simulink model "State_Feedback_Linear_ROS"  (R2022b)
settings: Solver=FixedStepAuto  StartTime=0.0  StopTime=128  FixedStep=0.02  RelTol=1e-3
undefined symbols (not defined in the file): unicycle, X, Y
libraries: robotlib x3, simulink_extras x2
settings Model: PauseTimes=14.13  Creator=Musta  LastModifiedBy=mustacchim
settings OptimizationCC: EnhancedBackFolding=on  PassReuseOutputArgsAs=Individual arguments  ZeroExternalMemoryAtStartup=off  ZeroInternalMemoryAtStartup=off  MaxStackSize=64  OptimizeBlockOrder=speed  DifferentSizesBufferReuse=on  OptimizationCustomize=off  EfficientTunableParamExpr=on
settings DebuggingCC: ParameterTunabilityLossMsg=error
settings HardwareCC: ProdBitPerPointer=32  ProdBitPerSizeT=32  ProdBitPerPtrDiffT=32  ProdLargestAtomicFloat=None  ProdIntDivRoundTo=Undefined  ProdEndianess=Unspecified  ProdWordSize=32  ProdHWDeviceType=Generic->Unspecified (assume 32-bit Generic)
settings SFSimCC: MATLABDynamicMemAlloc=off
settings RTWCC: Description=Embedded Coder  SystemTargetFile=ert.tlc  HardwareBoard=Robot Operating System (ROS)  TLCOptions="-aInlineSetEventsForThisBaseRateFcn=TLC_FALSE -aSuppressMultiTaskScheduler=TLC_FALSE  -aRateBasedStepFcn=0"  TemplateMakefile=ert_default_tmf  Toolchain=Catkin  TargetLang=C++
settings CodeAppCC: ForceParamTrailComments=on  IgnoreCustomStorageClasses=off  OperatorAnnotations=on  SimulinkDataObjDesc=on  SFDataObjDesc=on  InsertBlockDesc=on

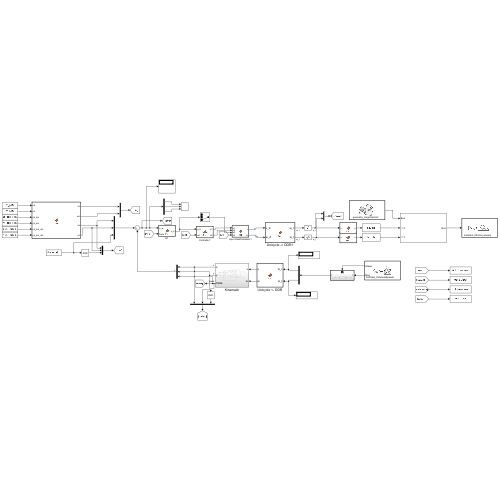
[thumbnail: Simulink's stored preview of the top-level diagram]
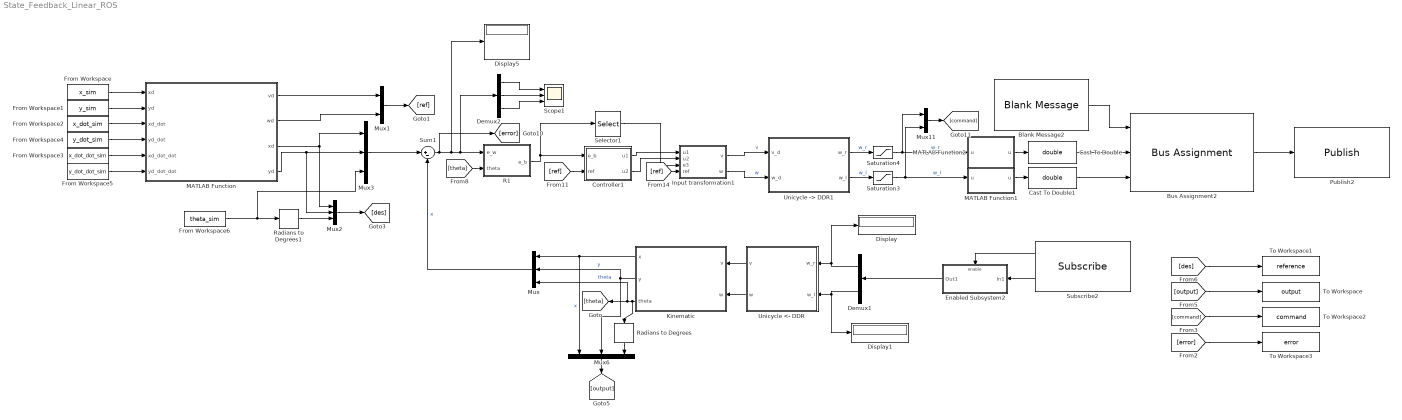
== system State_Feedback_Linear_ROS ==
  Blank Message2 : robotlib/Blank Message  messageClass=Message  entityType=geometry_msgs/Vector3  messageType=geometry_msgs/Vector3  SampleTime=0.02  legacyBusStruct=off
      settings: LibrarySourceBlock=roslib/ROS/Blank Message
  Bus Assignment2 : BusAssignment  AssignedSignals=X,Y
  Cast To Double : DataTypeConversion  OutDataTypeStr=double  SaturateOnIntegerOverflow=off  RndMeth=Floor
  Cast To Double1 : DataTypeConversion  OutDataTypeStr=double  SaturateOnIntegerOverflow=off  RndMeth=Floor
  Controller1 : MATLAB Function  TreatAsAtomicUnit=on
  Demux1 : Demux  Outputs=2
  Demux2 : Demux  Outputs=3
  Display : Display
  Display1 : Display
  Display5 : Display
  Enabled Subsystem2 : Subsystem  TreatAsAtomicUnit=on
  From Workspace : FromWorkspace  VariableName=x_sim
  From Workspace1 : FromWorkspace  VariableName=y_sim
  From Workspace2 : FromWorkspace  VariableName=x_dot_sim
  From Workspace3 : FromWorkspace  VariableName=x_dot_dot_sim
  From Workspace4 : FromWorkspace  VariableName=y_dot_sim
  From Workspace5 : FromWorkspace  VariableName=y_dot_dot_sim
  From Workspace6 : FromWorkspace  VariableName=theta_sim
  Input transformation1 : MATLAB Function  TreatAsAtomicUnit=on
  Kinematic : Subsystem
  MATLAB Function : MATLAB Function  TreatAsAtomicUnit=on
  MATLAB Function1 : MATLAB Function  TreatAsAtomicUnit=on
  MATLAB Function2 : MATLAB Function  TreatAsAtomicUnit=on
  Mux{,2..3,6} (4 alike) : Mux  Inputs=3
  Mux1 : Mux  Inputs=2
  Mux11 : Mux  Inputs=2
  Publish2 : robotlib/Publish  topicSource=Select from ROS network  topic=/turtlebot_03/cmd_wheels  messageType=geometry_msgs/Vector3  legacyBusStruct=off  messageQueueLength=1
      settings: LibrarySourceBlock=roslib/ROS/Publish
  R1 : MATLAB Function  TreatAsAtomicUnit=on
  Radians to Degrees : simulink_extras/Transformations/Radians to Degrees
  Radians to Degrees1 : simulink_extras/Transformations/Radians to Degrees
  Saturation3 : Saturate  UpperLimit=8  LowerLimit=-8
  Saturation4 : Saturate  UpperLimit=8  LowerLimit=-8
  Scope1 : Scope  NumInputPorts=3
  Selector1 : Selector  InputPortWidth=3  IndexOptions=Index vector (dialog)  Indices=3  OutputSizes=1
  Subscribe2 : robotlib/Subscribe  topicSource=Select from ROS network  topic=/turtlebot_03/wheelSpeeds  messageType=geometry_msgs/Vector3  SampleTime=0.02  legacyBusStruct=off  messageQueueLength=1
      settings: LibrarySourceBlock=roslib/ROS/Subscribe
  Sum1 : Sum  Inputs=|+-
  To Workspace : ToWorkspace  VariableName=output  SaveFormat=Structure With Time  SampleTime=-1
  To Workspace1 : ToWorkspace  VariableName=reference  SaveFormat=Structure With Time  SampleTime=-1
  To Workspace2 : ToWorkspace  VariableName=command  SaveFormat=Structure With Time  SampleTime=-1
  To Workspace3 : ToWorkspace  VariableName=error  SaveFormat=Structure With Time  SampleTime=-1
  "Unicycle -> DDR1" : MATLAB Function  TreatAsAtomicUnit=on
  Unicycle <- DDR : MATLAB Function  TreatAsAtomicUnit=on
  wires:
  [des] -> To Workspace1/1
  [output] -> To Workspace/1
  [command] -> To Workspace2/1
  [error] -> To Workspace3/1
  Demux2/3 -> Scope1/3
  Input transformation1/2(w) -> "Unicycle -> DDR1"/2(w_d)  "w"
  "Unicycle -> DDR1"/2(w_l) -> Saturation3/1  "w_l"
  Sum1/1 -> [error], Display5/1, R1/1(e_w), Demux2/1
  Demux2/1 -> Scope1/1
  "Unicycle -> DDR1"/1(w_r) -> Saturation4/1  "w_r"
  Input transformation1/1(v) -> "Unicycle -> DDR1"/1(v_d)  "v"
  Bus Assignment2/1 -> Publish2/1
  Blank Message2/1 -> Bus Assignment2/1
  Mux11/1 -> [command]
  Selector1/1 -> Input transformation1/3(e3)
  Controller1/1(u1) -> Input transformation1/1(u1)
  [theta] -> R1/2(theta)
  [ref] -> Controller1/2(ref)
  [ref] -> Input transformation1/4(ref)
  R1/1(e_b) -> Selector1/1, Controller1/1(e_b)
  Saturation4/1 -> MATLAB Function2/1("u "), Mux11/1  "w_r"
  Saturation3/1 -> MATLAB Function1/1("u "), Mux11/2  "w_l"
  Controller1/2(u2) -> Input transformation1/2(u2)
  Demux2/2 -> Scope1/2
  Mux/1 -> Sum1/2  "x"
  From Workspace/1 -> MATLAB Function/1("xd ")
  From Workspace6/1 -> Radians to Degrees1/1, Mux3/3
  Mux2/1 -> [des]
  Mux1/1 -> [ref]
  MATLAB Function/2(wd) -> Mux1/2
  From Workspace1/1 -> MATLAB Function/2("yd ")
  From Workspace3/1 -> MATLAB Function/5(xd_dot_dot)
  From Workspace5/1 -> MATLAB Function/6(yd_dot_dot)
  MATLAB Function/4(yd) -> Mux2/2, Mux3/2
  From Workspace2/1 -> MATLAB Function/3(xd_dot)
  From Workspace4/1 -> MATLAB Function/4(yd_dot)
  MATLAB Function/1(vd) -> Mux1/1
  Mux3/1 -> Sum1/1
  Radians to Degrees1/1 -> Mux2/3
  MATLAB Function/3(xd) -> Mux3/1, Mux2/1
  Demux1/1 -> Display/1, Unicycle <- DDR/1(w_r)
  Enabled Subsystem2/1(Out1) -> Demux1/1
  Radians to Degrees/1 -> Mux6/3
  Unicycle <- DDR/1(v) -> Kinematic/1(v)
  Mux6/1 -> [output]
  Kinematic/3(theta) -> Mux/3, [theta], Radians to Degrees/1  "theta"
  Demux1/2 -> Display1/1, Unicycle <- DDR/2(w_l)
  Kinematic/1(x) -> Mux/1, Mux6/1  "x"
  Subscribe2/1 -> Enabled Subsystem2/Enable
  Kinematic/2(y) -> Mux/2, Mux6/2  "y"
  Unicycle <- DDR/2(w) -> Kinematic/2(w)
  Subscribe2/2 -> Enabled Subsystem2/1(In1)
  MATLAB Function2/1(u) -> Cast To Double/1
  MATLAB Function1/1(u) -> Cast To Double1/1
  Cast To Double/1 -> Bus Assignment2/2
  Cast To Double1/1 -> Bus Assignment2/3

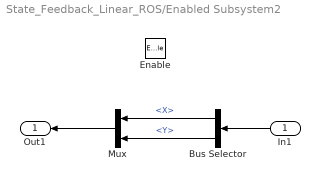
== system State_Feedback_Linear_ROS/Enabled Subsystem2 ==
  In1 : Inport
  Enable : EnablePort
  Bus Selector : BusSelector  OutputSignals=X,Y
  Mux : Mux  Inputs=2
  Out1 : Outport
  wires:
  Mux/1 -> Out1/1
  Bus Selector/1 -> Mux/1  "<X>"
  Bus Selector/2 -> Mux/2  "<Y>"
  In1/1 -> Bus Selector/1

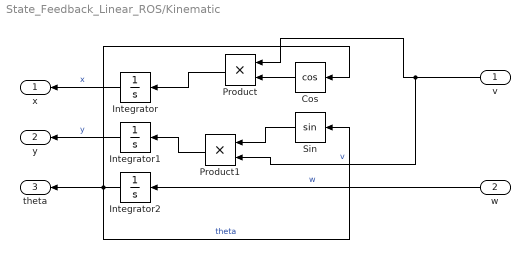
== system State_Feedback_Linear_ROS/Kinematic ==
  v : Inport
  w : Inport  Port=2
  Cos : Trigonometry  Operator=cos
  Integrator : Integrator  InitialCondition=unicycle.ic.x
  Integrator1 : Integrator  InitialCondition=unicycle.ic.y
  Integrator2 : Integrator  InitialCondition=unicycle.ic.theta
  Product : Product
  Product1 : Product
  Sin : Trigonometry
  x : Outport
  y : Outport  Port=2
  theta : Outport  Port=3
  wires:
  w/1 -> Integrator2/1  "w"
  Product/1 -> Integrator/1
  v/1 -> Product/1, Product1/2  "v"
  Cos/1 -> Product/2
  Integrator1/1 -> y/1  "y"
  Integrator/1 -> x/1  "x"
  Integrator2/1 -> theta/1, Sin/1, Cos/1  "theta"
  Product1/1 -> Integrator1/1
  Sin/1 -> Product1/1

== matlab function State_Feedback_Linear_ROS/MATLAB Function1 ==
  data: u input; u output
function u = fcn(u)


    if (isnan(u))
        u = 0.1;
    end

end

== matlab function State_Feedback_Linear_ROS/MATLAB Function ==
  data: xd input; vd output; yd input; xd_dot input; yd_dot input; xd_dot_dot input; yd_dot_dot input; wd output; xd output; yd output
function [vd, wd, xd, yd] = fcn(xd, yd, xd_dot, yd_dot, xd_dot_dot, yd_dot_dot)
    
    vd = sqrt(xd_dot.^2 + yd_dot.^2);
    wd = (xd_dot.*yd_dot_dot - xd_dot_dot.*yd_dot) / (xd_dot.^2 + yd_dot.^2);

    xd = xd;
    yd = yd;

end

== matlab function State_Feedback_Linear_ROS/MATLAB Function2 ==
  data: u input; u output
function u = fcn(u)

    if (isnan(u))
        u = 0.1;
    end

end

== matlab function State_Feedback_Linear_ROS/Controller1 ==
  data: e_b input; u1 output; ref input; u2 output
function [u1,u2] = fcn(e_b, ref)

    %#codegen
    coder.extrinsic('evalin')
    a = 0;                  % Needed in order to set variable class correctly
    zeta = 0;                  % Needed in order to set variable class correctly
    a = evalin('base','a'); % Read value from workspace
    zeta = evalin('base','zeta'); % Read value from workspace

    k1 = 2*zeta*a;
    k2 = (a^2 - ref(2)^2) / ref(1);
    k3 = 2*zeta*a;

    u1 = -k1*e_b(1);
    u2 = -k2*e_b(2) -k3*e_b(3);

end

== matlab function State_Feedback_Linear_ROS/Input transformation1 ==
  data: u1 input; v output; u2 input; e3 input; w output; ref input
function [v, w] = fcn(u1, u2, e3, ref)

    v = ref(1)*cos(e3) - u1;
    w = ref(2) - u2;

end

== matlab function State_Feedback_Linear_ROS/Unicycle <- DDR ==
  data: w_r input; v output; w_l input; w output
function [v, w] = fcn(w_r, w_l)

    %#codegen
    coder.extrinsic('evalin')
    d = 0;                  % Needed in order to set variable class correctly
    r = 0;                  % Needed in order to set variable class correctly
    d = evalin('base','unicycle.d'); % Read value from workspace
    r = evalin('base','unicycle.r'); % Read value from workspace

    v = r*(w_r + w_l)/2; % rad/s
    w = r*(w_r - w_l)/d; % rad/s

end

== matlab function State_Feedback_Linear_ROS/R1 ==
  data: e_w input; e_b output; theta input
function e_b  = fcn(e_w, theta)
    
    R = [cos(theta), sin(theta), 0;
        -sin(theta), cos(theta), 0;
         0, 0, 1];

    e_b = R * e_w;

end

== matlab function State_Feedback_Linear_ROS/Unicycle -> DDR1 ==
  data: v_d input; w_r output; w_d input; w_l output
function [w_r, w_l] = fcn(v_d, w_d)

    %#codegen
    coder.extrinsic('evalin')
    d = 0;                  % Needed in order to set variable class correctly
    r = 0;                  % Needed in order to set variable class correctly
    d = evalin('base','unicycle.d'); % Read value from workspace
    r = evalin('base','unicycle.r'); % Read value from workspace

    w_r = ((2 * v_d) + (w_d * d)) / (2 * r);
    w_l = ((2 * v_d) - (w_d * d)) / (2 * r);

end
